simulink model "nimbus"  (R2015b)
settings: Solver=FixedStepDiscrete  SolverMode=SingleTasking  StartTime=0.0  StopTime=sim_stop_time  FixedStep=sim_time_step_size  RelTol=1e-3
PreLoadFcn:
  | nimbus_bus_all;
values from neighbouring files (symbols this model uses):
  sim_time_step_size = 1/100    (= 0.01)    [nimbus_sim_init.m]
undefined symbols (not defined in the file or in its folder): accel, cam_cam1_lander_dcm, cam_cam1_lander_quat, cam_cam1_pos_in_lander, cam_processing_delay_cycles, central_body_flattening, central_body_radius, central_body_rotation_rate, csc_ekf_nonlinear_filter_lib, csc_ekf_nonlinear_filter_new, csc_est_state_est_new, csc_estimation_lib, csc_kfl_kalman_filter_lib, csc_kfl_kalman_filter_new, csc_ldr_flir_lidar, csc_ldr_flir_lidar_lib, csc_rsp_radar_sensor_prep_lib, csc_rsp_radar_sensor_prep_new, csc_sensors_a, csc_sensors_lib_a, csc_sim_simulation, csc_sim_simulation_lib, csc_snp_sensor_prep_lib, csc_snp_sensor_prep_new, csci_fsw, csci_fsw_lib, csci_gsse, csci_gsse_lib, est_time_step, fcv_initializing, ini_alt_wrt_meanrad, ini_epoch_seconds, kfl_lidar_switch_altitude, kfl_use_range_meas, ldr_lander_dcm, ldr_use_meme_flag, pwr_ldr_on_state, q, snp_dtheta_filter_coeffs, snp_dtheta_filter_order, snp_meas_noise_alt, snp_meas_noise_angle, snp_meas_noise_angle_exp, snp_meas_noise_angle_gain, snp_meas_noise_dtheta, snp_meas_noise_dtheta_exp, snp_meas_noise_dtheta_gain, snp_meas_noise_indep, snp_R_lower_limit_alt, snp_R_lower_limit_angle, snp_R_lower_limit_dtheta, snp_rdr_index, snp_rdr_zero_index, snp_zero_index, snp_zero_meas, swm_num_switches, x
undefined symbols (not defined in the file): ldr_position_in_lander
libraries: util_common_lib x23, util_info_lib x13, simulink x8, util_frame_rotation_lib x5, util_quat_lib x5, simulink_extras x4, util_geodesy_lib x2, csu_cfe_cfe_time_lib x2, csu_tlm_telemetry_lib x2, csu_flr_lidar_noise_model_lib x2, csc_act_actuator_manager_lib x1, csc_cmp_command_mode_process_lib x1
(part 2 of 2)

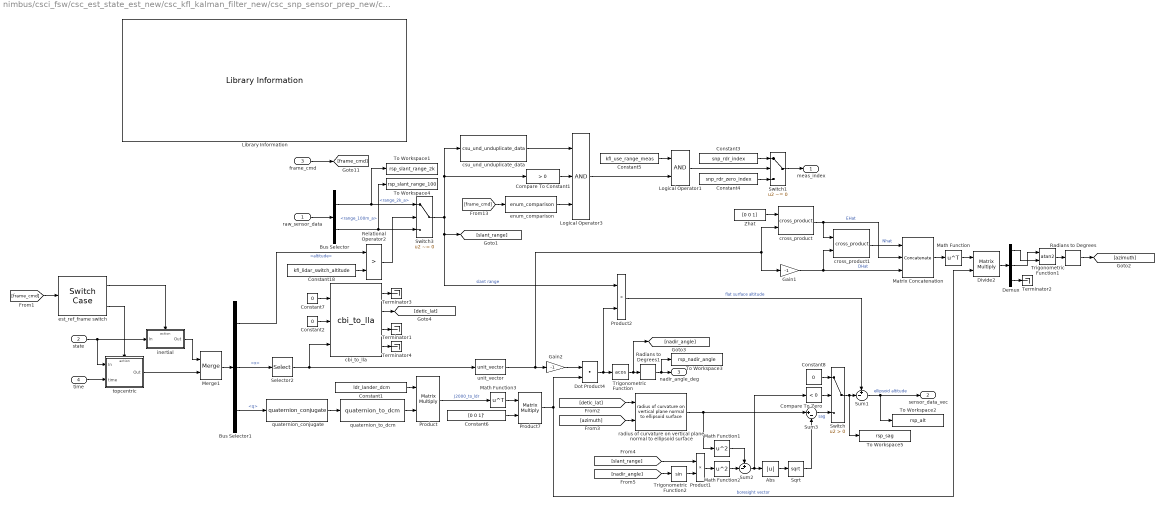
== system nimbus/csci_fsw/csc_est_state_est_new/csc_kfl_kalman_filter_new/csc_snp_sensor_prep_new/csc_rsp_radar_sensor_prep_new ==
  raw_sensor_data : Inport
  state : Inport  Port=2
  frame_cmd : Inport  Port=3
  time : Inport  Port=4
  Abs : Abs
  Bus Selector : BusSelector  OutputSignals=range_2k_a,range_100m_a
  Bus Selector1 : BusSelector  OutputSignals=altitude,x,q
  Compare To Constant1 : simulink/Logic and Bit Operations/Compare To Constant  relop=>  const=0  OutDataTypeStr=uint8
  Compare To Zero : simulink/Logic and Bit Operations/Compare To Zero  relop=<  OutDataTypeStr=boolean
  Constant1 : Constant  Value=ldr_lander_dcm
  Constant18 : Constant  Value=kfl_lidar_switch_altitude
  Constant2 : Constant  Value=0
  Constant3 : Constant  Value=snp_rdr_index
  Constant4 : Constant  Value=snp_rdr_zero_index
  Constant5 : Constant  Value=kfl_use_range_meas
  Constant6 : Constant  Value=[0 0 1]'  VectorParams1D=off
  Constant7 : Constant  Value=0
  Constant8 : Constant  Value=0
  Demux : Demux  Outputs=3
  Divide2 : Product  Inputs=**  Multiplication=Matrix(*)
  Dot Product4 : DotProduct  InputSameDT=on  OutDataTypeStr=Inherit: Inherit via internal rule
  Gain1 : Gain  Gain=-1
  Gain2 : Gain  Gain=-1
  Library Information : util_info_lib/Library Information  owner='NONE'
  Logical Operator1 : Logic  AllPortsSameDT=off  OutDataTypeStr=boolean
  Logical Operator3 : Logic  Inputs=3  AllPortsSameDT=off  OutDataTypeStr=boolean
  Math Function : Math  Operator=transpose  SaturateOnIntegerOverflow=on
  Math Function1 : Math  Operator=square  SaturateOnIntegerOverflow=on
  Math Function2 : Math  Operator=square  SaturateOnIntegerOverflow=on
  Math Function3 : Math  Operator=transpose  SaturateOnIntegerOverflow=on
  Matrix Concatenation : Concatenate  NumInputs=3  Mode=Multidimensional array  ConcatenateDimension=2
  Merge1 : Merge  InitialOutput=0
  Product : Product  Multiplication=Matrix(*)  RndMeth=Zero
  Product1 : Product  Inputs=**  RndMeth=Zero
  Product2 : Product  Inputs=**  RndMeth=Zero
  Product7 : Product  Multiplication=Matrix(*)  RndMeth=Zero
  Radians to Degrees : simulink_extras/Transformations/Radians to Degrees
  Radians to Degrees1 : simulink_extras/Transformations/Radians to Degrees
  Relational Operator2 : RelationalOperator  Operator=>  OutDataTypeStr=boolean
  Selector2 : Selector  InputPortWidth=kfl_n_state  IndexOptions=Index vector (dialog)  Indices=kfl_pos_index  OutputSizes=1
  Sqrt : Sqrt  SaturateOnIntegerOverflow=on
  Sum1 : Sum  Inputs=+-|
  Sum2 : Sum  Inputs=+-|  AccumDataTypeStr=double
  Sum3 : Sum  Inputs=|+-
  Switch : Switch  Criteria=u2 > Threshold
  Switch1 : Switch  Criteria=u2 ~= 0
  Switch3 : Switch  Criteria=u2 ~= 0
  Terminator{1..4} (4 alike) : Terminator
  To Workspace1 : ToWorkspace  VariableName=rsp_slant_range_2k  SaveFormat=Structure With Time  SampleTime=-1
  To Workspace2 : ToWorkspace  VariableName=rsp_alt  SaveFormat=Structure With Time  SampleTime=-1
  To Workspace3 : ToWorkspace  VariableName=rsp_nadir_angle  SaveFormat=Structure With Time  SampleTime=-1
  To Workspace4 : ToWorkspace  VariableName=rsp_slant_range_100  SaveFormat=Structure With Time  SampleTime=-1
  To Workspace5 : ToWorkspace  VariableName=rsp_sag  SaveFormat=Structure With Time  SampleTime=-1
  Trigonometric Function : Trigonometry  Operator=acos
  Trigonometric Function1 : Trigonometry  Operator=atan2
  Trigonometric Function2 : Trigonometry
  Zhat : Constant  Value=[0 0 1]
  cbi_to_lla : util_frame_rotation_lib/cbi_to_lla  a=central_body_radius  b=central_body_radius*(1-central_body_flattening)  omega=central_body_rotation_rate(3)
  cross_product : util_common_lib/cross_product  SystemSampleTime=-1
  cross_product1 : util_common_lib/cross_product  SystemSampleTime=-1
  csu_und_unduplicate_data : csu_und_unduplicate_lib/csu_und_unduplicate_data  initial_compare=0
  enum_comparison : util_common_lib/enum_comparison  comparison_type===
  est_ref_frame switch : SwitchCase  CaseConditions={uint8(enum_reference_frame.inertial),uint8(enum_reference_frame.topocentric)}  ShowDefaultCase=off
  inertial : Subsystem  TreatAsAtomicUnit=on
  quaternion_conjugate : util_quat_lib/quaternion_conjugate  SystemSampleTime=-1
  quaternion_to_dcm : util_quat_lib/quaternion_to_dcm  SystemSampleTime=-1
  radius of curvature on vertical plane normal to ellipsoid surface : util_geodesy_lib/radius of curvature on vertical plane normal to ellipsoid surface  a=central_body_radius  b=central_body_radius*(1-central_body_flattening)
  topcentric : Subsystem  TreatAsAtomicUnit=on
  unit_vector : util_common_lib/unit_vector  SystemSampleTime=-1
  meas_index : Outport
  sensor_data_vec : Outport  Port=2
  nadir_angle_deg : Outport  Port=3
  wires:
  enum_comparison/1 -> Logical Operator3/3
  Switch1/1 -> meas_index/1
  raw_sensor_data/1 -> Bus Selector/1
  Compare To Constant1/1 -> Logical Operator3/2
  Bus Selector1/2 -> Selector2/1  "<x>"
  Bus Selector1/3 -> quaternion_conjugate/1  "<q>"
  Bus Selector1/1 -> Relational Operator2/1  "<altitude>"
  Relational Operator2/1 -> Switch3/2
  Bus Selector/1 -> To Workspace1/1, Switch3/1  "<range_2k_a>"
  Bus Selector/2 -> To Workspace4/1, Switch3/3  "<range_100m_a>"
  Switch3/1 -> Product2/1, [slant_range], Compare To Constant1/1, csu_und_unduplicate_data/1  "slant range"
  Constant3/1 -> Switch1/1
  Constant4/1 -> Switch1/3
  Logical Operator3/1 -> Logical Operator1/2
  Logical Operator1/1 -> Switch1/2
  Constant5/1 -> Logical Operator1/1
  Selector2/1 -> cbi_to_lla/3, unit_vector/1
  Product/1 -> Math Function3/1  "J2000_to_ldr"
  Math Function3/1 -> Product7/1
  quaternion_to_dcm/1 -> Product/2
  Constant1/1 -> Product/1
  Constant6/1 -> Product7/2
  quaternion_conjugate/1 -> quaternion_to_dcm/1
  Gain2/1 -> Dot Product4/1
  Dot Product4/1 -> Product2/2, Trigonometric Function/1
  Trigonometric Function/1 -> [nadir_angle], Radians to Degrees1/1
  Radians to Degrees1/1 -> nadir_angle_deg/1, To Workspace3/1
  [frame_cmd] -> est_ref_frame switch/1
  est_ref_frame switch/1 -> inertial/Action
  state/1 -> topcentric/1(In), inertial/1(In)
  inertial/1(Out) -> Merge1/1
  topcentric/1(Out) -> Merge1/2
  est_ref_frame switch/2 -> topcentric/Action
  time/1 -> topcentric/2(time)
  Merge1/1 -> Bus Selector1/1
  frame_cmd/1 -> [frame_cmd]
  [frame_cmd] -> enum_comparison/1
  Product2/1 -> Sum1/1  "flat surface altitude"
  Constant18/1 -> Relational Operator2/2
  csu_und_unduplicate_data/1 -> Logical Operator3/1
  Demux/2 -> Trigonometric Function1/1
  Demux/1 -> Trigonometric Function1/2
  Trigonometric Function1/1 -> Radians to Degrees/1
  Demux/3 -> Terminator2/1
  Divide2/1 -> Demux/1
  Math Function/1 -> Divide2/1
  Zhat/1 -> cross_product/1
  unit_vector/1 -> cross_product/2, Gain1/1, Gain2/1
  Matrix Concatenation/1 -> Math Function/1
  cross_product1/1 -> Matrix Concatenation/1  "Nhat"
  cross_product/1 -> cross_product1/1, Matrix Concatenation/2  "EHat"
  Gain1/1 -> cross_product1/2, Matrix Concatenation/3  "DHat"
  [detic_lat] -> radius of curvature on vertical plane normal to ellipsoid surface/1
  [azimuth] -> radius of curvature on vertical plane normal to ellipsoid surface/2
  Product7/1 -> Dot Product4/2, Divide2/2  "boresight vector"
  Radians to Degrees/1 -> [azimuth]
  radius of curvature on vertical plane normal to ellipsoid surface/1 -> Sum3/1, Math Function1/1
  Math Function1/1 -> Sum2/1
  Math Function2/1 -> Sum2/2
  Sqrt/1 -> Sum3/2
  [nadir_angle] -> Trigonometric Function2/1
  Trigonometric Function2/1 -> Product1/2
  Product1/1 -> Math Function2/1
  [slant_range] -> Product1/1
  Sum1/1 -> To Workspace2/1, sensor_data_vec/1  "ellipsoid altitude"
  Sum3/1 -> Switch/3  "sag"
  cbi_to_lla/2 -> [detic_lat]
  Constant2/1 -> cbi_to_lla/2
  Constant7/1 -> cbi_to_lla/1
  cbi_to_lla/3 -> Terminator1/1
  cbi_to_lla/1 -> Terminator3/1
  cbi_to_lla/4 -> Terminator4/1
  Compare To Zero/1 -> Switch/2
  Constant8/1 -> Switch/1
  Abs/1 -> Sqrt/1
  Sum2/1 -> Abs/1, Compare To Zero/1
  Switch/1 -> To Workspace5/1, Sum1/2

== system nimbus/csci_gsse/csc_sim_simulation/csc_sensors_a/csc_ldr_flir_lidar/csc_lpr_short_long_range_pair_a ==
  env_metric : Inport
  time : Inport  Port=2
  Library Information : util_info_lib/Library Information  owner='escrane'
  csu_flr_lidar_noise_model_100ma : csu_flr_lidar_noise_model_lib/csu_flr_lidar_noise_model  model_type=flr_100m_model
  csu_flr_lidar_noise_model_2ka : csu_flr_lidar_noise_model_lib/csu_flr_lidar_noise_model  model_type=flr_2k_model
  csu_rng_range_model_100ma : csu_rng_range_model_lib/csu_rng_range_model  position_in_lander=ldr_position_in_lander  lander_dcm=ldr_lander_dcm
  csu_rng_range_model_2ka : Subsystem  AncestorBlock=csu_rng_range_model_lib/csu_rng_range_model  SystemSampleTime=0.1  mask{position_in_lander=ldr_position_in_lander, lander_dcm=ldr_lander_dcm}
      mask prompts: position_in_lander "LIDAR Position in Body Frame (meters)"; lander_dcm "LIDAR Attitude wrt Body Frame (DCM)"
  lower_rate : util_common_lib/lower_rate  counter_max=flr_2k_rate_counter  counter_init=0
  lower_rate1 : util_common_lib/lower_rate  counter_max=flr_100m_rate_counter  counter_init=0
  range_2k : Outport
  range_100m : Outport  Port=2
  wires:
  csu_flr_lidar_noise_model_2ka/1 -> lower_rate/1
  csu_rng_range_model_2ka/1(slant_range) -> csu_flr_lidar_noise_model_2ka/1
  lower_rate/1 -> range_2k/1  "range_2k"
  env_metric/1 -> csu_rng_range_model_100ma/1, csu_rng_range_model_2ka/1(env_metric)
  csu_flr_lidar_noise_model_100ma/1 -> lower_rate1/1
  csu_rng_range_model_100ma/1 -> csu_flr_lidar_noise_model_100ma/1
  lower_rate1/1 -> range_100m/1  "range_100m"
  [time] -> csu_rng_range_model_2ka/2(time)
  time/1 -> [time]
  [time] -> csu_rng_range_model_100ma/2

== system nimbus/csci_fsw/csc_est_state_est_new/csc_kfl_kalman_filter_new/csc_snp_sensor_prep_new/csc_rsp_radar_sensor_prep_new/inertial ==
  In : Inport
  Action Port : ActionPort  ActionType=case
  Signal Conversion : SignalConversion
  Out : Outport
  wires:
  In/1 -> Signal Conversion/1
  Signal Conversion/1 -> Out/1

== system nimbus/csci_fsw/csc_est_state_est_new/csc_kfl_kalman_filter_new/csc_snp_sensor_prep_new/csc_rsp_radar_sensor_prep_new/topcentric ==
  In : Inport
  time : Inport  Port=2
  Action Port : ActionPort  ActionType=case
  Bus Selector1 : BusSelector  OutputSignals=x,accel,q
  BusAssignment : BusAssignment  AssignedSignals=x,accel,q
  Selector1 : Selector  InputPortWidth=kfl_n_state  IndexOptions=Index vector (dialog)  Indices=kfl_vel_index  OutputSizes=1
  Selector3 : Selector  InputPortWidth=kfl_n_state  IndexOptions=Index vector (dialog)  Indices=kfl_pos_index  OutputSizes=1
  Signal Conversion : SignalConversion
  assign_pos : Assignment  IndexOptions=Index vector (dialog)  Indices=kfl_pos_index  OutputSizes=1
  assign_vel : Assignment  IndexOptions=Index vector (dialog)  Indices=kfl_vel_index  OutputSizes=1
  quaternions_only : util_frame_rotation_lib/quaternions_only  SystemSampleTime=-1
  state_topocentric_to_inertial : util_fsw_frame_rotation_lib/state_topocentric_to_inertial  SystemSampleTime=-1
  Out : Outport
  wires:
  state_topocentric_to_inertial/3 -> BusAssignment/3
  state_topocentric_to_inertial/4 -> BusAssignment/4
  BusAssignment/1 -> Out/1
  time/1 -> quaternions_only/1
  quaternions_only/1 -> state_topocentric_to_inertial/5
  quaternions_only/2 -> state_topocentric_to_inertial/6
  Bus Selector1/1 -> assign_pos/1, Selector3/1, Selector1/1  "<x>"
  Selector3/1 -> state_topocentric_to_inertial/1
  Selector1/1 -> state_topocentric_to_inertial/2
  Bus Selector1/2 -> state_topocentric_to_inertial/3  "<accel>"
  Bus Selector1/3 -> state_topocentric_to_inertial/4  "<q>"
  state_topocentric_to_inertial/1 -> assign_pos/2
  assign_pos/1 -> assign_vel/1
  state_topocentric_to_inertial/2 -> assign_vel/2
  assign_vel/1 -> BusAssignment/2
  In/1 -> Signal Conversion/1
  Signal Conversion/1 -> BusAssignment/1, Bus Selector1/1

== system nimbus/csci_gsse/csc_sim_simulation/csc_sensors_a/csc_ldr_flir_lidar/csc_lpr_short_long_range_pair_a/csu_rng_range_model_2ka ==
  env_metric : Inport
  time : Inport  Port=2
  Bus Selector : BusSelector  OutputSignals=lander_state_bus.rtk_pos_eci,lander_state_bus.rrk_q_body_from_eci
  Constant : Constant  Value=position_in_lander
  Constant1 : Constant  Value=lander_dcm
  Constant2 : Constant  Value=ldr_use_meme_flag
  Constant3 : Constant  Value=-1
  Constant4 : Constant  Value=[0 0 1]'  VectorParams1D=off
  Library Information : util_info_lib/Library Information  owner='NONE'
  Math Function3 : Math  Operator=transpose  SaturateOnIntegerOverflow=on
  Product : Product  Multiplication=Matrix(*)  RndMeth=Zero
  Product7 : Product  Multiplication=Matrix(*)  RndMeth=Zero
  Sum3 : Sum  Inputs=|++
  Switch1 : Switch  Criteria=u2 ~= 0  InputSameDT=on
  Terminator1 : Terminator
  Terminator2 : Terminator
  quaternion_conjugate : util_quat_lib/quaternion_conjugate  SystemSampleTime=-1
  quaternion_rotation2 : util_quat_lib/quaternion_rotation  SystemSampleTime=-1
  quaternion_to_dcm : util_quat_lib/quaternion_to_dcm  SystemSampleTime=-1
  slant range to surface with workspace output : Subsystem  AncestorBlock=util_geodesy_lib/slant range to surface with workspace output
  slant_range : Outport
  wires:
  Constant3/1 -> Switch1/1
  Constant2/1 -> Switch1/2
  slant range to surface with workspace output/2(ellipsoid) -> Switch1/3
  Switch1/1 -> slant_range/1
  Bus Selector/2 -> quaternion_conjugate/1, quaternion_rotation2/2  "<rrk_q_body_from_eci>"
  Bus Selector/1 -> Sum3/1  "<rtk_pos_eci>"
  env_metric/1 -> Bus Selector/1
  quaternion_rotation2/1 -> Sum3/2
  Constant/1 -> quaternion_rotation2/1
  slant range to surface with workspace output/1(flat) -> Terminator1/1
  time/1 -> Terminator2/1
  Product/1 -> Math Function3/1  "J2000_to_ldr"
  Math Function3/1 -> Product7/1
  quaternion_to_dcm/1 -> Product/2
  Constant1/1 -> Product/1
  Constant4/1 -> Product7/2
  quaternion_conjugate/1 -> quaternion_to_dcm/1
  Sum3/1 -> slant range to surface with workspace output/1(pos_inertial)  "T"
  Product7/1 -> slant range to surface with workspace output/2(boresight_inertial)

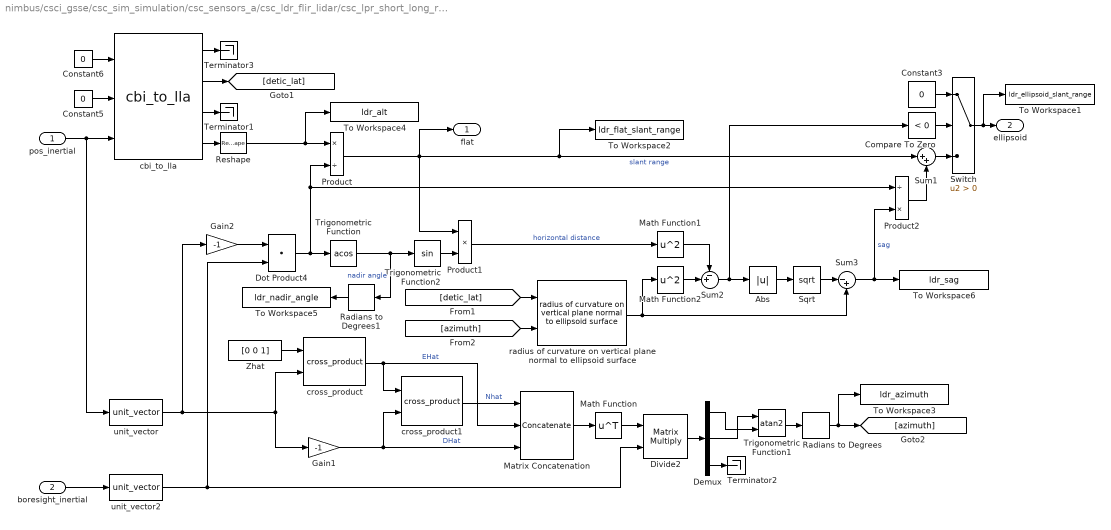
== system nimbus/csci_gsse/csc_sim_simulation/csc_sensors_a/csc_ldr_flir_lidar/csc_lpr_short_long_range_pair_a/csu_rng_range_model_2ka/slant range to surface with workspace output ==
  pos_inertial : Inport
  boresight_inertial : Inport  Port=2
  Abs : Abs
  Compare To Zero : simulink/Logic and Bit Operations/Compare To Zero  relop=<  OutDataTypeStr=boolean
  Constant3 : Constant  Value=0
  Constant5 : Constant  Value=0
  Constant6 : Constant  Value=0
  Demux : Demux  Outputs=3
  Divide2 : Product  Inputs=**  Multiplication=Matrix(*)
  Dot Product4 : DotProduct  InputSameDT=on  OutDataTypeStr=Inherit: Inherit via internal rule
  Gain1 : Gain  Gain=-1
  Gain2 : Gain  Gain=-1
  Math Function : Math  Operator=transpose  SaturateOnIntegerOverflow=on
  Math Function1 : Math  Operator=square  SaturateOnIntegerOverflow=on
  Math Function2 : Math  Operator=square  SaturateOnIntegerOverflow=on
  Matrix Concatenation : Concatenate  NumInputs=3  Mode=Multidimensional array  ConcatenateDimension=2
  Product : Product  Inputs=*/  RndMeth=Zero
  Product1 : Product  Inputs=**  RndMeth=Zero
  Product2 : Product  Inputs=/*  RndMeth=Zero
  Radians to Degrees : simulink_extras/Transformations/Radians to Degrees
  Radians to Degrees1 : simulink_extras/Transformations/Radians to Degrees
  Reshape : Reshape
  Sqrt : Sqrt  SaturateOnIntegerOverflow=on
  Sum1 : Sum  Inputs=|++  AccumDataTypeStr=double
  Sum2 : Sum  Inputs=-+|  AccumDataTypeStr=double
  Sum3 : Sum  Inputs=|-+  AccumDataTypeStr=double
  Switch : Switch  Criteria=u2 > Threshold
  Terminator1 : Terminator
  Terminator2 : Terminator
  Terminator3 : Terminator
  To Workspace1 : ToWorkspace  VariableName=ldr_ellipsoid_slant_range  SaveFormat=Structure With Time  SampleTime=-1
  To Workspace2 : ToWorkspace  VariableName=ldr_flat_slant_range  SaveFormat=Structure With Time  SampleTime=-1
  To Workspace3 : ToWorkspace  VariableName=ldr_azimuth  SaveFormat=Structure With Time  SampleTime=-1
  To Workspace4 : ToWorkspace  VariableName=ldr_alt  SaveFormat=Structure With Time  SampleTime=-1
  To Workspace5 : ToWorkspace  VariableName=ldr_nadir_angle  SaveFormat=Structure With Time  SampleTime=-1
  To Workspace6 : ToWorkspace  VariableName=ldr_sag  SaveFormat=Structure With Time  SampleTime=-1
  Trigonometric Function : Trigonometry  Operator=acos
  Trigonometric Function1 : Trigonometry  Operator=atan2
  Trigonometric Function2 : Trigonometry
  Zhat : Constant  Value=[0 0 1]
  cbi_to_lla : util_frame_rotation_lib/cbi_to_lla  a=central_body_radius  b=central_body_radius*(1-central_body_flattening)  omega=central_body_rotation_rate(3)
  cross_product : util_common_lib/cross_product  SystemSampleTime=-1
  cross_product1 : util_common_lib/cross_product  SystemSampleTime=-1
  radius of curvature on vertical plane normal to ellipsoid surface : util_geodesy_lib/radius of curvature on vertical plane normal to ellipsoid surface  a=central_body_radius  b=central_body_radius*(1-central_body_flattening)
  unit_vector : util_common_lib/unit_vector  SystemSampleTime=-1
  unit_vector2 : util_common_lib/unit_vector  SystemSampleTime=-1
  flat : Outport
  ellipsoid : Outport  Port=2
  wires:
  Switch/1 -> ellipsoid/1, To Workspace1/1
  Sum1/1 -> Switch/3
  Product2/1 -> Sum1/2
  Dot Product4/1 -> Trigonometric Function/1, Product/2, Product2/1
  Sqrt/1 -> Sum3/1
  Math Function1/1 -> Sum2/1
  Math Function2/1 -> Sum2/2
  radius of curvature on vertical plane normal to ellipsoid surface/1 -> Sum3/2, Math Function2/1
  Product1/1 -> Math Function1/1  "horizontal distance"
  Product/1 -> Product1/1, Sum1/1, To Workspace2/1, flat/1  "slant range"
  Trigonometric Function2/1 -> Product1/2
  Trigonometric Function/1 -> Radians to Degrees1/1, Trigonometric Function2/1  "nadir angle"
  Demux/2 -> Trigonometric Function1/1
  Demux/1 -> Trigonometric Function1/2
  Trigonometric Function1/1 -> Radians to Degrees/1
  Demux/3 -> Terminator2/1
  Divide2/1 -> Demux/1
  Math Function/1 -> Divide2/1
  Zhat/1 -> cross_product/1
  unit_vector/1 -> Gain2/1, cross_product/2, Gain1/1
  Matrix Concatenation/1 -> Math Function/1
  cross_product1/1 -> Matrix Concatenation/1  "Nhat"
  cross_product/1 -> cross_product1/1, Matrix Concatenation/2  "EHat"
  Gain1/1 -> cross_product1/2, Matrix Concatenation/3  "DHat"
  [detic_lat] -> radius of curvature on vertical plane normal to ellipsoid surface/1
  cbi_to_lla/2 -> [detic_lat]
  cbi_to_lla/4 -> Reshape/1
  boresight_inertial/1 -> unit_vector2/1
  pos_inertial/1 -> cbi_to_lla/3, unit_vector/1
  Constant5/1 -> cbi_to_lla/2
  Constant6/1 -> cbi_to_lla/1
  cbi_to_lla/3 -> Terminator1/1
  cbi_to_lla/1 -> Terminator3/1
  Gain2/1 -> Dot Product4/1
  [azimuth] -> radius of curvature on vertical plane normal to ellipsoid surface/2
  Sum2/1 -> Abs/1, Compare To Zero/1
  unit_vector2/1 -> Dot Product4/2, Divide2/2
  Abs/1 -> Sqrt/1
  Compare To Zero/1 -> Switch/2
  Constant3/1 -> Switch/1
  Sum3/1 -> To Workspace6/1, Product2/2  "sag"
  Radians to Degrees1/1 -> To Workspace5/1
  Reshape/1 -> To Workspace4/1, Product/1
  Radians to Degrees/1 -> To Workspace3/1, [azimuth]
